simulink model "abs_model"  (R2012b)
settings: Solver=ode45  StartTime=0.0  StopTime=10.0  RelTol=1e-3
settings Model: Creator=inteco  LastModifiedBy=inteco
settings DataIOCC: SignalLoggingSaveFormat=ModelDataLogs
settings DebuggingCC: SaveWithParameterizedLinksMsg=none  SignalResolutionControl=TryResolveAllWithWarning  SolverPrmCheckMsg=none  MultiTaskDSMMsg=warning  MultiTaskCondExecSysMsg=none  FcnCallInpInsideContextMsg=UseLocalSettings  StrictBusMsg=None
settings HardwareCC: TargetUnknown=on
settings RTWCC: IncludeERTFirstTime=on
settings GRTTargetCC: CombineOutputUpdateFcns=off  GRTInterface=on

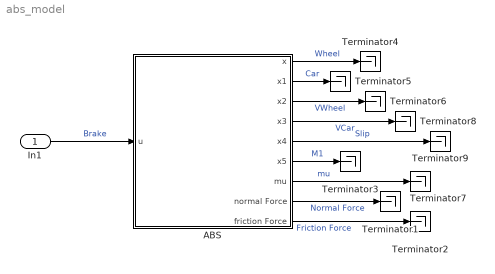
== system abs_model ==
  In1 : Inport
  ABS : Subsystem  mask{r=[99.5 99]*1e-3, J=[7.5281 25.603]*1e-3, d=[1.2 2.25]*1e-4, M=[3  93]*1e-3, Mg=19.6181, w=[-0.04240011450454   0.00000000029375   0.03508217905067   0.40662691102315], p=2.09945271667129, a=0.00025724985785, L=0.370, phi=65.61*pi/180, uu=[0.40748031496063 15.24 -6.21], tau=0.048, xini=[180 180 0]}
      mask prompts: r "r1, r2"; J "J1, J2"; d "d1, d2"; M "M10, M20"; uu "brake param. u0, b1 b2"; tau "tau (c31=1/tau)"; xini "xini = [x1(0) x2(0) x3(0)]"
      mask init:
      | J1 = J(1);J2 = J(2);d1 = d(1);d2=d(2);r1 = r(1);r2=r(2);M10 = M(1);M20 = M(2);u0 = uu(1);b1 = uu(2);b2=uu(3);
      mask Display: plot([-0.2 -0.2], [-0.2 -0.2], [1.2 1.2], [1.2 1.2], [0.9 0.9], [0.6 0.9], [0.9 0.9], [0.3 0.5], [0.85 0.85 0.95 0.95], [0.7 0.5 0.5 0.7], [0.75 0.75], [0.8 0.9], [0.75 0.75], [0.3 0.4], [0.75 0.775], [0.4 0.425], [0.775 0.725 0.775], [0.425 0.475 0.525], [0.775 0.725 0.775], [0.525 0.575 0.625], [0.775 0.725 0.775], [0.625 0.675 0.725], [0.775 0.725 0.75], [0.725 0.775 0.8], [0.65 0.95], [0.9 0.9], [0.65 0.7], [0.9 1], [0.7 0.75], [0.9 1], [0.75 0.8], [0.9 1], [0.8 0.85], [0.9 1], [0.85 0.9], [0.9 1], [0.9 0.95], [0.9 1], [0.95 1], [0.9 1], 0.4+0.3*sin([0 0.20 0.41 0.62 0.83 1.04 1.25 1.46 1.67 1.88 2.09 2.30 2.51 2.72 2.93 3.14 3.35 3.56 3.76 3.97 4.18 4.39 4.60 4.81 5.02 5.23 5.44 5.65 5.86 6.07 6.28]), 0.3+0.3*cos([0 0.20 0.41 0.62 0.83 1.04 1.25 1.46 1.67 1.88 2.09 2.30 2.51 2.72 2.93 3.14 3.35 3.56 3.76 3.97 4.18 4.39 4.60 4.81 5.02 5.23 5.44 5.65 5.86 6.07 6.28]), (1-0.005)+0.005*sin([0 0.20 0.41 0.62 0.83 1.04 1.25 1.46 1.67 1.88 2.09 2.30 2.51 2.72 2.93 3.14 3.35 3.56 3.76 3.97 4.18 4.39 4.60 4.81 5.02 5.23 5.44 5.65 5.86 6.07 6.28]), 0.3+0.005*cos([0 0.20 0.41 0.62 0.83 1.04 1.25 1.46 1.67 1.88 2.09 2.30 2.51 2.72 2.93 3.14 3.35 3.56 3.76 3.97 4.18 4.39 4.60 4.81 5.02 5.23 5.44 5.65 5.86 6.07 6.28]), 0.4+0.005*sin([0 0.20 0.41 0.62 0.83 1.04 1.25 1.46 1.67 1.88 2.09 2.30 2.51 2.72 2.93 3.14 3.35 3.56 3.76 3.97 4.18 4.39 4.60 4.81 5.02 5.23 5.44 5.65 5.86 6.07 6.28]), 0.3+0.005*cos([0 0.20 0.41 0.62 0.83 1.04 1.25 1.46 1.67 1.88 2.09 2.30 2.51 2.72 2.93 3.14 3.35 3.56 3.76 3.97 4.18 4.39 4.60 4.81 5.02 5.23 5.44 5.65 5.86 6.07 6.28]), [0.4 1], [0.3 0.3], [0 1], [0 0] )
  Terminator{1..9} (9 alike) : Terminator
  wires:
  ABS/1(x) -> Terminator4/1  "Wheel"
  ABS/2(x1) -> Terminator5/1  "Car"
  ABS/3(x2) -> Terminator6/1  "VWheel"
  ABS/5(x4) -> Terminator9/1  "Slip"
  ABS/7(mu) -> Terminator7/1  "mu"
  ABS/8(normal Force) -> Terminator1/1  "Normal Force"
  ABS/9(friction Force) -> Terminator2/1  "Friction Force"
  ABS/4(x3) -> Terminator8/1  "VCar"
  ABS/6(x5) -> Terminator3/1  "M1"
  In1/1 -> ABS/1(u)  "Brake"

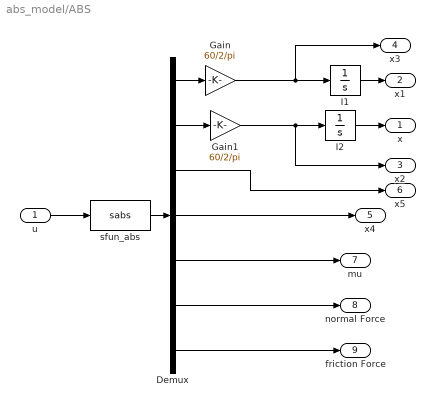
== system abs_model/ABS ==
  u : Inport
  Demux : Demux  Outputs=7
  Gain : Gain  Gain=60/2/pi  SaturateOnIntegerOverflow=on  OutDataTypeStr=Inherit: Same as input  ParamDataTypeStr=Inherit: Same as input
  Gain1 : Gain  Gain=60/2/pi  SaturateOnIntegerOverflow=on  OutDataTypeStr=Inherit: Same as input  ParamDataTypeStr=Inherit: Same as input
  I1 : Integrator
  I2 : Integrator
  sfun_abs : S-Function  FunctionName=sabs  Parameters=r1,r2,J1,J2,d1,d2,M10,M20,Mg,w,p,a,L,phi,u0,b1,b2,tau,xini  EnableBusSupport=off
  x : Outport
  x1 : Outport  Port=2
  x2 : Outport  Port=3
  x3 : Outport  Port=4
  x4 : Outport  Port=5
  x5 : Outport  Port=6
  mu : Outport  Port=7
  normal Force : Outport  Port=8
  friction Force : Outport  Port=9
  wires:
  u/1 -> sfun_abs/1
  sfun_abs/1 -> Demux/1
  Demux/1 -> Gain/1
  Gain/1 -> I1/1, x3/1
  Demux/2 -> Gain1/1
  Gain1/1 -> I2/1, x2/1
  I1/1 -> x1/1
  I2/1 -> x/1
  Demux/4 -> x4/1
  Demux/3 -> x5/1
  Demux/5 -> mu/1
  Demux/6 -> normal Force/1
  Demux/7 -> friction Force/1
